simulink subsystem "IdealTrans_MotionSensor"  (R2025a)
settings: Solver=VariableStepAuto  StartTime=0.0  StopTime=10.0  RelTol=1e-3
model mask{ns_sw=0, ns_pw=0, ts=-1, init_pos=0}
  mask prompts: ns_sw "noise_switch [1 = on, 0 = off]"; ns_pw "noise_power [mm²/Hz]"; ts "sample_time [s]"; init_pos "init_pos [mm]"
libraries: fl_lib x2, simulink x1, nesl_utility x1
settings Model: Creator=CelestialAurora  LastModifiedBy=CelestialAurora

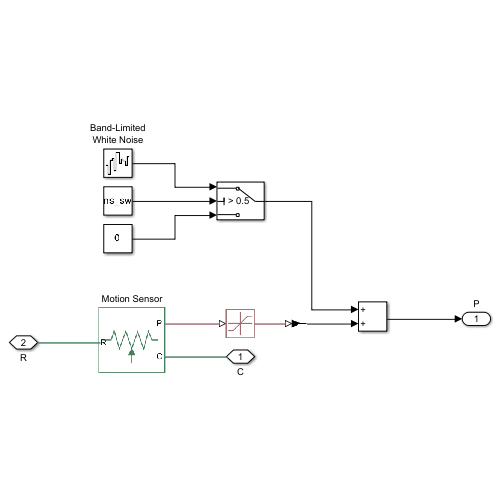
[thumbnail: Simulink's stored preview of the top-level diagram]
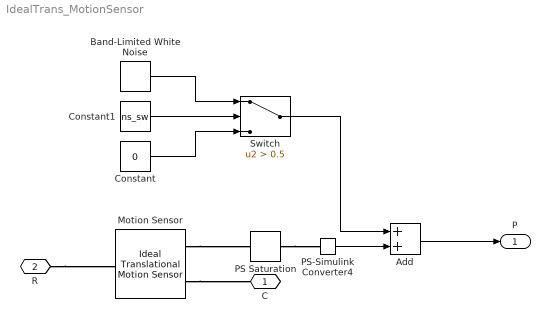
== system IdealTrans_MotionSensor ==
  Add : Sum
  Band-Limited White Noise : simulink/Sources/Band-Limited White Noise  Cov=ns_pw  Ts=ts  seed=[23341]
  Constant : Constant  Value=0
  Constant1 : Constant  Value=ns_sw
  Motion Sensor : fl_lib/Mechanical/Mechanical Sensors/Ideal Translational Motion Sensor  reference=foundation.enum.MeasurementReference.difference  acceleration_port=false  velocity_port=false  position_port=true  offset=init_pos mm
      settings: InternalSimscapePortConfiguration="{\"Bottom\":[],\"Left\":[{\"id\":\"R\",\"label\":\"R\",\"type\":\"foundation.mechanical.translational.translational\"}],\"Right\":[{\"id\":\"C\",\"label\":\"C\",\"type\":\"foundation.mechanical.translational.translational\"},{\"id\":\"P\",\"label\":\"P\",\"type\":\"output\"}],\"Top\":[]}"
  PS Saturation : fl_lib/Physical Signals/Nonlinear Operators/PS Saturation  upper_limit=10 mm  lower_limit=0 mm  ZeroCross=true
  PS-Simulink Converter4 : nesl_utility/PS-Simulink Converter  PhysicalDomain=network_engine_domain  SubClassName=ps_output  LeftPortType=input  RightPortType=output  PseudoPeriodic=off  Frequencies=[]  VectorFormat=inherit  Unit=mm  AffineConversion=on
  Switch : Switch  Criteria=u2 > Threshold  Threshold=0.5  SaturateOnIntegerOverflow=off  InputSameDT=off
  C : PMIOPort  Side=Left
  R : PMIOPort  Port=2  Side=Left
  P : Outport
  wires:
  Constant/1 -> Switch/3
  Add/1 -> P/1
  Switch/1 -> Add/1
  Band-Limited White Noise/1 -> Switch/1
  PS-Simulink Converter4/1 -> Add/2
  Constant1/1 -> Switch/2
  connections:
  R/RConn1 -- Motion Sensor/LConn1
  PS Saturation/RConn1 -- PS-Simulink Converter4/LConn1
  Motion Sensor/RConn1 -- C/RConn1
  Motion Sensor/RConn2 -- PS Saturation/LConn1
